simulink model "Cphi"  (R2024a)
settings: Solver=VariableStepAuto  StartTime=0.0  StopTime=7  RelTol=1e-3
values from neighbouring files (symbols this model uses):
  K = 0.38    [RunCphi.m]    (also in RunCrho.m = 0.07; RunGphi.m; RunGrho.m = 0.07; RunPhi.m)
  Kp = 1    [RunCphi.m]    (also in RunCrho.m = 28; RunPhi.m = 20; RunRho.m = 28; Runmotor_control.m = 2.8)
  sigma = 8.5    [RunCphi.m]    (also in RunCrho.m = 11; RunGphi.m; RunGrho.m = 11; RunPhi.m)
libraries: simulink x1
settings Model: Creator=sansh  LastModifiedBy=liama
settings SolverCC: AlgebraicLoopSolver=TrustRegion
settings DataIOCC: ReturnWorkspaceOutputs=off
settings DebuggingCC: UnconnectedInputMsg=warning  UnconnectedOutputMsg=warning  UnconnectedLineMsg=warning  ArithmeticOperatorsInVariantConditions=warning
settings ModelReferenceCC: EnableRefExpFcnMdlSchedulingChecks=on
settings SFSimCC: SimUseLocalCustomCode=off  CustomCodeUndefinedFunction=UseInterfaceOnly
settings RTWCC: RTWUseLocalCustomCode=off  GPUComputeCapability=3.5
settings CodeAppCC: StateflowObjectComments=on

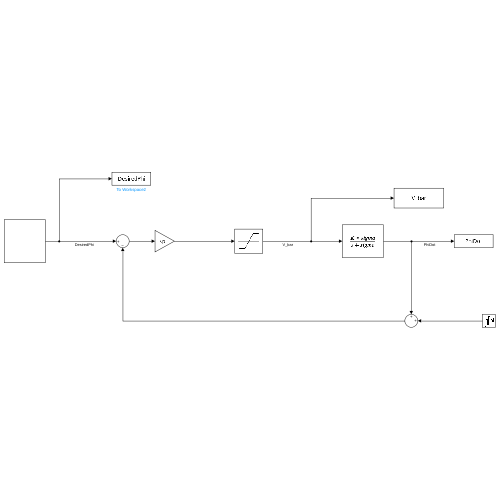
[thumbnail: Simulink's stored preview of the top-level diagram]
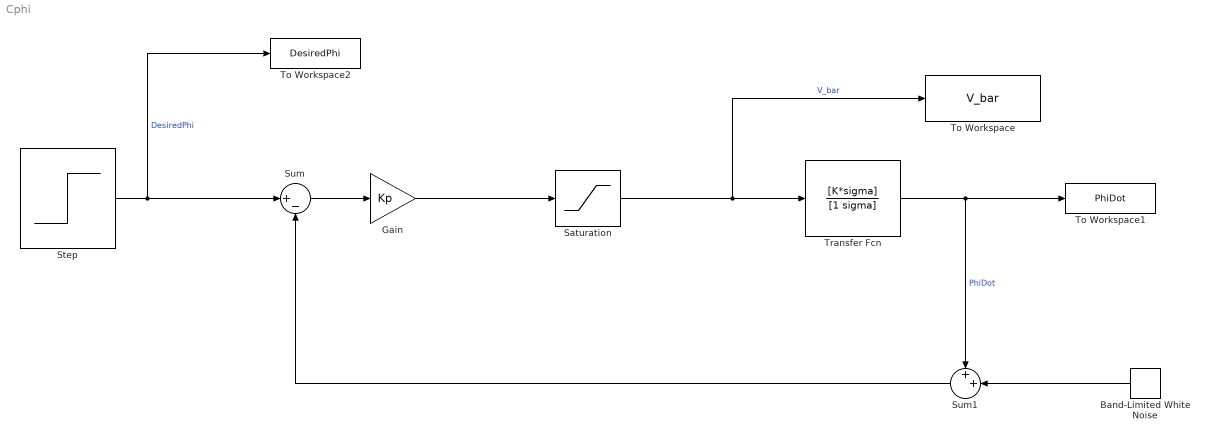
== system Cphi ==
  Band-Limited White Noise : simulink/Sources/Band-Limited White Noise  Cov=[0.1]  Ts=0.1  seed=[23341]
  Gain : Gain  Gain=Kp
  Saturation : Saturate
  Step : Step  SampleTime=0
  Sum : Sum  Inputs=|+-
  Sum1 : Sum  Inputs=++|
  To Workspace : ToWorkspace  VariableName=V_bar  SaveFormat=Timeseries  SampleTime=-1
  To Workspace1 : ToWorkspace  VariableName=PhiDot  SaveFormat=Timeseries  SampleTime=-1
  To Workspace2 : ToWorkspace  VariableName=DesiredPhi  SaveFormat=Timeseries  SampleTime=-1
  Transfer Fcn : TransferFcn  Numerator=[K*sigma]  Denominator=[1 sigma]
  wires:
  Saturation/1 -> To Workspace/1, Transfer Fcn/1  "V_bar"
  Transfer Fcn/1 -> Sum1/1, To Workspace1/1  "PhiDot"
  Gain/1 -> Saturation/1
  Sum/1 -> Gain/1
  Sum1/1 -> Sum/2
  Band-Limited White Noise/1 -> Sum1/2
  Step/1 -> To Workspace2/1, Sum/1  "DesiredPhi"
